simulink model "EPT"  (R2019b)
settings: Solver=FixedStepDiscrete  StartTime=0.0  StopTime=5  FixedStep=0.005  RelTol=1e-3  EnableMultiTasking=on
PreLoadFcn:
  | try, model_open; catch, disp('Error occurred while executing model pre-load callback: model_open.m'); disp('Please assure that the MATLAB working directory is set to the model directory before opening.'); end
InitFcn:
  | try, model_open; catch, end
undefined symbols (not defined in the file or in its folder): Bridge, GCM, H, ln, raptor_get_param_eval, raptor_get_safe_string, raptor_xcp_function
libraries: Raptor_lib x2810, simulink x374, hdlsllib x19
(part 19 of 45)

== system EPT/Foreground_TimeBase_5ms/CAN/CAN3_exec/HyPer9_MCU/TPDO6 ==
  Trigger : TriggerPort  VariantControl=Variant  PortDimensions=1
  Constant : Constant  Value=0.001  OutDataTypeStr=double
  Constant1 : Constant  Value=0.001  OutDataTypeStr=double
  Constant2 : Constant  Value=0.001  OutDataTypeStr=double
  Constant3 : Constant  Value=4  OutDataTypeStr=double
  Constant4 : Constant  Value=4  OutDataTypeStr=double
  Convert_Byte2Data : Subsystem
  Convert_Byte2Data1 : Subsystem
  Convert_Byte2Data2 : Subsystem
  Convert_Byte2Data3 : Subsystem
  Convert_Byte2Data4 : Subsystem
  Demux : Demux  Outputs=8
  raptor_can_rxraw : Raptor_lib/CAN/raptor_can_rxraw  canBus='CAN3'  extendedId=0  showAge=1  id=hex2dec('6A0')  idMask=hex2dec('1FFFFFFF')  mailbox=''  queueSize=1
      settings: SourceProductName=Raptor
  raptor_measurement1 : Raptor_lib/Data Storage/raptor_measurement  paramName='Meas_Motor2_Current'  nameSource=Parameter  calDispType=Number  calEnum={'False', 'True'}  calGain=1.0  calOffset=0.0  calMax=inf  calMin=-inf  calFormat='-1'  calUnit=''  calHelp=''  calAccess=1  calFunction=raptor_xcp_function(gcb)  calVisible=on
      settings: SourceProductName=Raptor
  raptor_measurement2 : Raptor_lib/Data Storage/raptor_measurement  paramName='Meas_Motor1_Current'  nameSource=Parameter  calDispType=Number  calEnum={'False', 'True'}  calGain=1.0  calOffset=0.0  calMax=inf  calMin=-inf  calFormat='-1'  calUnit=''  calHelp=''  calAccess=1  calFunction=raptor_xcp_function(gcb)  calVisible=on
      settings: SourceProductName=Raptor
  raptor_measurement3 : Raptor_lib/Data Storage/raptor_measurement  paramName='Meas_Driver_Output3_Current'  nameSource=Parameter  calDispType=Number  calEnum={'False', 'True'}  calGain=1.0  calOffset=0.0  calMax=inf  calMin=-inf  calFormat='-1'  calUnit=''  calHelp=''  calAccess=1  calFunction=raptor_xcp_function(gcb)  calVisible=on
      settings: SourceProductName=Raptor
  raptor_measurement4 : Raptor_lib/Data Storage/raptor_measurement  paramName='Meas_Driver_Output2_Current'  nameSource=Parameter  calDispType=Number  calEnum={'False', 'True'}  calGain=1.0  calOffset=0.0  calMax=inf  calMin=-inf  calFormat='-1'  calUnit=''  calHelp=''  calAccess=1  calFunction=raptor_xcp_function(gcb)  calVisible=on
      settings: SourceProductName=Raptor
  raptor_measurement5 : Raptor_lib/Data Storage/raptor_measurement  paramName='Meas_Driver_Output1_Current'  nameSource=Parameter  calDispType=Number  calEnum={'False', 'True'}  calGain=1.0  calOffset=0.0  calMax=inf  calMin=-inf  calFormat='-1'  calUnit=''  calHelp=''  calAccess=1  calFunction=raptor_xcp_function(gcb)  calVisible=on
      settings: SourceProductName=Raptor
  wires:
  Constant1/1 -> Convert_Byte2Data1/4(Factor)
  Constant/1 -> Convert_Byte2Data/4(Factor)
  Demux/3 -> Convert_Byte2Data1/1(LowByte)
  Demux/4 -> Convert_Byte2Data1/2(HighByte)
  Convert_Byte2Data1/1(Data) -> raptor_measurement4/1
  Convert_Byte2Data/1(Data) -> raptor_measurement5/1
  Demux/2 -> Convert_Byte2Data/2(HighByte)
  Demux/1 -> Convert_Byte2Data/1(LowByte)
  raptor_can_rxraw/5 -> Demux/1
  Convert_Byte2Data2/1(Data) -> raptor_measurement3/1
  Demux/6 -> Convert_Byte2Data2/2(HighByte)
  Demux/5 -> Convert_Byte2Data2/1(LowByte)
  Constant2/1 -> Convert_Byte2Data2/4(Factor)
  Convert_Byte2Data3/1(Data) -> raptor_measurement2/1
  Convert_Byte2Data4/1(Data) -> raptor_measurement1/1
  Demux/7 -> Convert_Byte2Data3/2(LowByte)
  Demux/8 -> Convert_Byte2Data4/2(LowByte)
  Constant3/1 -> Convert_Byte2Data3/3(Factor)
  Constant4/1 -> Convert_Byte2Data4/3(Factor)

== system EPT/Foreground_TimeBase_5ms/CAN/CAN3_exec/OBC/CountTrigger ==
  Counter : Inport
  Constant1 : Constant  Value=0
  Constant3 : Constant
  CycleTrigger : Subsystem
  Switch : Switch  Threshold=1
  Unit Delay : UnitDelay  SampleTime=-1  HasFrameUpgradeWarning=on
  Tirgger : Outport  VectorParamsAs1DForOutWhenUnconnected=off
  wires:
  Switch/1 -> CycleTrigger/1(In1)
  Constant3/1 -> Switch/3
  Constant1/1 -> Switch/1
  Counter/1 -> CycleTrigger/2(In2)
  CycleTrigger/1(Trigger) -> Tirgger/1, Unit Delay/1
  Unit Delay/1 -> Switch/2

== system EPT/Foreground_TimeBase_5ms/CAN/CAN3_exec/OBC/CountTrigger1 ==
  Counter : Inport
  Constant1 : Constant  Value=0
  Constant3 : Constant
  CycleTrigger : Subsystem
  Switch : Switch  Threshold=1
  Unit Delay : UnitDelay  SampleTime=-1  HasFrameUpgradeWarning=on
  Tirgger : Outport  VectorParamsAs1DForOutWhenUnconnected=off
  wires:
  Switch/1 -> CycleTrigger/1(In1)
  Constant3/1 -> Switch/3
  Constant1/1 -> Switch/1
  Counter/1 -> CycleTrigger/2(In2)
  CycleTrigger/1(Trigger) -> Tirgger/1, Unit Delay/1
  Unit Delay/1 -> Switch/2

== system EPT/Foreground_TimeBase_5ms/CAN/CAN3_exec/OBC/OBC ==
  Rx_Time : Inport
  Tx_Time : Inport  Port=2
  OBC_Rx : Subsystem
  OBC_Tx : Subsystem
  wires:
  Rx_Time/1 -> OBC_Rx/Trigger
  Tx_Time/1 -> OBC_Tx/Trigger

== system EPT/Foreground_TimeBase_5ms/CAN/CAN3_exec/PWCU_GENERATOR/CountTrigger ==
  Counter : Inport
  Constant1 : Constant  Value=0
  Constant3 : Constant
  CycleTrigger : Subsystem
  Switch : Switch  Threshold=1
  Unit Delay : UnitDelay  SampleTime=-1  HasFrameUpgradeWarning=on
  Tirgger : Outport  VectorParamsAs1DForOutWhenUnconnected=off
  wires:
  Unit Delay/1 -> Switch/2
  CycleTrigger/1(Trigger) -> Unit Delay/1, Tirgger/1
  Counter/1 -> CycleTrigger/2(In2)
  Constant1/1 -> Switch/1
  Constant3/1 -> Switch/3
  Switch/1 -> CycleTrigger/1(In1)

== system EPT/Foreground_TimeBase_5ms/CAN/CAN3_exec/PWCU_GENERATOR/CountTrigger1 ==
  Counter : Inport
  Constant1 : Constant  Value=0
  Constant3 : Constant
  CycleTrigger : Subsystem
  Switch : Switch  Threshold=1
  Unit Delay : UnitDelay  SampleTime=-1  HasFrameUpgradeWarning=on
  Tirgger : Outport  VectorParamsAs1DForOutWhenUnconnected=off
  wires:
  Unit Delay/1 -> Switch/2
  CycleTrigger/1(Trigger) -> Unit Delay/1, Tirgger/1
  Counter/1 -> CycleTrigger/2(In2)
  Constant1/1 -> Switch/1
  Constant3/1 -> Switch/3
  Switch/1 -> CycleTrigger/1(In1)

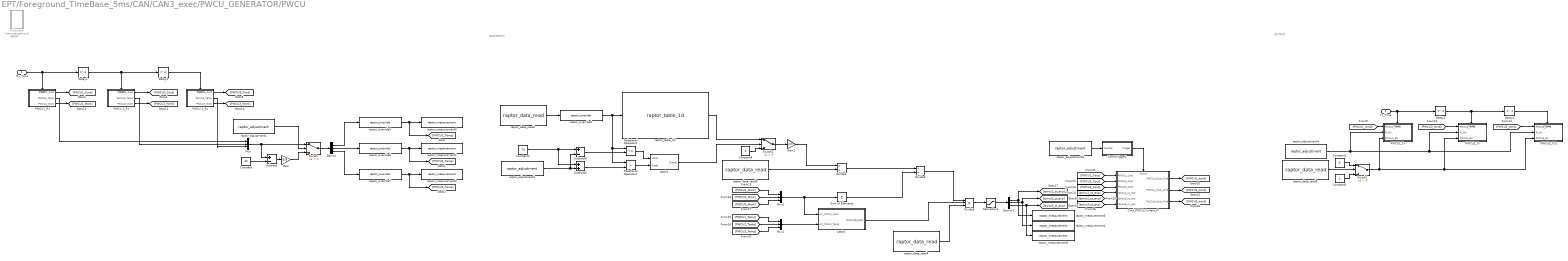
== system EPT/Foreground_TimeBase_5ms/CAN/CAN3_exec/PWCU_GENERATOR/PWCU ==
  note: INPUT
  note: OUTPUT
  note: Applictation
  Rx_Time : Inport
  Tx_Time : Inport  Port=2
  "Cmd_PWCU_Current_PI " : Subsystem
  Constant : Constant  Value=32
  Constant1 : Constant  Value=0
  Constant2 : Constant  Value=70
  Constant3 : Constant
  Constant4 : Constant  Value=0
  CountTrigger1 : Subsystem
  Delay{1..4} (4 alike) : Delay  DelayLength=1
  Demux : Demux  Outputs=3
  Demux1 : Demux  Outputs=3
  Divide3 : Product  Inputs=*/
  Divide4 : Product  Inputs=*/
  Divide5 : Product  Inputs=***
  Gain : Gain  Gain=5/9
  Gain1 : Gain  Gain=1000
  Latch1 : Subsystem
  Latch2 : Subsystem
  Mux : Mux  Inputs=3
  Mux1 : Mux  Inputs=3
  Mux2 : Mux  Inputs=3
  PWCU 2_Rx : Subsystem
  PWCU 3_Rx : Subsystem
  PWCU1_Rx : Subsystem
  PWCU1_Tx : Subsystem
  PWCU2_Tx : Subsystem
  PWCU3_Tx3 : Subsystem
  Relational Operator2 : RelationalOperator  Operator=>  OutDataTypeStr=boolean  RndMeth=Simplest
  Relational Operator4 : RelationalOperator  Operator=<=  OutDataTypeStr=boolean  RndMeth=Simplest
  Saturation1 : Saturate  UpperLimit=20  LowerLimit=0
  Subsystem : Subsystem  Commented=on
  Subtract : Sum  Inputs=+-
  Subtract5 : Sum
  Subtract6 : Sum  Inputs=+-
  Sum of Elements : Sum  Inputs=+
  Switch : Switch  Criteria=u2 > Threshold
  Switch1 : Switch  Criteria=u2 > Threshold
  Switch2 : Switch  Criteria=u2 > Threshold
  raptor_adjustment1 : Raptor_lib/Data Storage/raptor_adjustment  paramName='Cal_Degree_Celsius'  nameSource=Parameter  initValue=0  dataType=boolean  storage=Calibration  calDispType=Number  calEnum={'False', 'True'}  calGain=1.0  calOffset=0.0  calMax=inf  calMin=-inf  calFormat='-1'  calUnit=''  calHelp=''  calAccess=1  calFunction=raptor_xcp_function(gcb)  calDispHeaders=off  calColHeaders={'Col1' 'Col2' 'Col3'}  calRowHeaders={'Row1' 'Row2' 'Row3'}
      settings: SourceProductName=Raptor
  raptor_adjustment16 : Raptor_lib/Data Storage/raptor_adjustment  paramName='PWCU_PI_Time'  nameSource=Parameter  initValue=30  dataType=double  storage=Calibration  calDispType=Number  calEnum={'False', 'True'}  calGain=1.0  calOffset=0.0  calMax=inf  calMin=-inf  calFormat='-1'  calUnit=''  calHelp=''  calAccess=1  calFunction=raptor_xcp_function(gcb)  calDispHeaders=off  calColHeaders={'Col1' 'Col2' 'Col3'}  calRowHeaders={'Row1' 'Row2' 'Row3'}
      settings: SourceProductName=Raptor
  raptor_adjustment2 : Raptor_lib/Data Storage/raptor_adjustment  paramName='Cal_RSOC_GENERATOR_Limit_error'  nameSource=Parameter  initValue=1  dataType=double  storage=Calibration  calDispType=Number  calEnum={'False', 'True'}  calGain=1.0  calOffset=0.0  calMax=inf  calMin=-inf  calFormat='-1'  calUnit=''  calHelp=''  calAccess=1  calFunction=raptor_xcp_function(gcb)  calDispHeaders=off  calColHeaders={'Col1' 'Col2' 'Col3'}  calRowHeaders={'Row1' 'Row2' 'Row3'}
      settings: SourceProductName=Raptor
  raptor_adjustment4 : Raptor_lib/Data Storage/raptor_adjustment  paramName='Cal_SWU_PI_On'  nameSource=Parameter  initValue=1  dataType=boolean  storage=Calibration  calDispType=Number  calEnum={'False', 'True'}  calGain=1.0  calOffset=0.0  calMax=inf  calMin=-inf  calFormat='-1'  calUnit=''  calHelp=''  calAccess=1  calFunction=raptor_xcp_function(gcb)  calDispHeaders=off  calColHeaders={'Col1' 'Col2' 'Col3'}  calRowHeaders={'Row1' 'Row2' 'Row3'}
      settings: SourceProductName=Raptor
  raptor_data_read3 : Raptor_lib/Data Storage/raptor_data_read  dataName='EPT_BPOBU_SOC'  dataShape=Scalar  idxSource=Input  idxRow=1  idxCol=1
      settings: SourceProductName=Raptor
  raptor_data_read4 : Raptor_lib/Data Storage/raptor_data_read  dataName='Ft_CHG_Vcell'  dataShape=Scalar  idxSource=Input  idxRow=1  idxCol=1
      settings: SourceProductName=Raptor
  raptor_data_read5 : Raptor_lib/Data Storage/raptor_data_read  dataName='EPT_HV_BUS_VOLT'  dataShape=Scalar  idxSource=Input  idxRow=1  idxCol=1
      settings: SourceProductName=Raptor
  raptor_data_read8 : Raptor_lib/Data Storage/raptor_data_read  dataName='Relay_BMS_SWU'  dataShape=Scalar  idxSource=Input  idxRow=1  idxCol=1
      settings: SourceProductName=Raptor
  raptor_measurement1 : Raptor_lib/Data Storage/raptor_measurement  paramName='Read_PWCU2_Temp'  nameSource=Parameter  calDispType=Number  calEnum={'False', 'True'}  calGain=1.0  calOffset=0.0  calMax=inf  calMin=-inf  calFormat='-1'  calUnit=''  calHelp=''  calAccess=1  calFunction=raptor_xcp_function(gcb)  calVisible=on
      settings: SourceProductName=Raptor
  raptor_measurement2 : Raptor_lib/Data Storage/raptor_measurement  paramName='Read_PWCU3_Temp'  nameSource=Parameter  calDispType=Number  calEnum={'False', 'True'}  calGain=1.0  calOffset=0.0  calMax=inf  calMin=-inf  calFormat='-1'  calUnit=''  calHelp=''  calAccess=1  calFunction=raptor_xcp_function(gcb)  calVisible=on
      settings: SourceProductName=Raptor
  raptor_measurement3 : Raptor_lib/Data Storage/raptor_measurement  paramName='Ipwcu3_cc_exp'  nameSource=Parameter  calDispType=Number  calEnum={'False', 'True'}  calGain=1.0  calOffset=0.0  calMax=inf  calMin=-inf  calFormat='-1'  calUnit=''  calHelp=''  calAccess=1  calFunction=raptor_xcp_function(gcb)  calVisible=on
      settings: SourceProductName=Raptor
  raptor_measurement4 : Raptor_lib/Data Storage/raptor_measurement  paramName='Ipwcu2_cc_exp'  nameSource=Parameter  calDispType=Number  calEnum={'False', 'True'}  calGain=1.0  calOffset=0.0  calMax=inf  calMin=-inf  calFormat='-1'  calUnit=''  calHelp=''  calAccess=1  calFunction=raptor_xcp_function(gcb)  calVisible=on
      settings: SourceProductName=Raptor
  raptor_measurement5 : Raptor_lib/Data Storage/raptor_measurement  paramName='Ipwcu1_cc_exp'  nameSource=Parameter  calDispType=Number  calEnum={'False', 'True'}  calGain=1.0  calOffset=0.0  calMax=inf  calMin=-inf  calFormat='-1'  calUnit=''  calHelp=''  calAccess=1  calFunction=raptor_xcp_function(gcb)  calVisible=on
      settings: SourceProductName=Raptor
  raptor_measurement6 : Raptor_lib/Data Storage/raptor_measurement  paramName='Read_PWCU1_Temp'  nameSource=Parameter  calDispType=Number  calEnum={'False', 'True'}  calGain=1.0  calOffset=0.0  calMax=inf  calMin=-inf  calFormat='-1'  calUnit=''  calHelp=''  calAccess=1  calFunction=raptor_xcp_function(gcb)  calVisible=on
      settings: SourceProductName=Raptor
  raptor_override4 : Raptor_lib/Data Storage/raptor_override  paramName='Cal_PWCU_EPT_BPOBU_SOC'  nameSource=Parameter  measurement=None  calDispType=Number  calEnum={'False', 'True'}  calGain=1.0  calOffset=0.0  calMax=inf  calMin=-inf  calFormat='-1'  calUnit=''  calHelp=''  calAccess=1  calFunction=[raptor_xcp_function(gcb) '|' raptor_get_param_eval(gcb, 'paramName') '_Override']
      settings: SourceProductName=Raptor
  raptor_override5 : Raptor_lib/Data Storage/raptor_override  paramName='Cal_PWCU1_Temp'  nameSource=Parameter  measurement=None  calDispType=Number  calEnum={'False', 'True'}  calGain=1.0  calOffset=0.0  calMax=inf  calMin=-inf  calFormat='-1'  calUnit=''  calHelp=''  calAccess=1  calFunction=[raptor_xcp_function(gcb) '|' raptor_get_param_eval(gcb, 'paramName') '_Override']
      settings: SourceProductName=Raptor
  raptor_override6 : Raptor_lib/Data Storage/raptor_override  paramName='Cal_PWCU2_Temp'  nameSource=Parameter  measurement=None  calDispType=Number  calEnum={'False', 'True'}  calGain=1.0  calOffset=0.0  calMax=inf  calMin=-inf  calFormat='-1'  calUnit=''  calHelp=''  calAccess=1  calFunction=[raptor_xcp_function(gcb) '|' raptor_get_param_eval(gcb, 'paramName') '_Override']
      settings: SourceProductName=Raptor
  raptor_override7 : Raptor_lib/Data Storage/raptor_override  paramName='Cal_PWCU3_Temp'  nameSource=Parameter  measurement=None  calDispType=Number  calEnum={'False', 'True'}  calGain=1.0  calOffset=0.0  calMax=inf  calMin=-inf  calFormat='-1'  calUnit=''  calHelp=''  calAccess=1  calFunction=[raptor_xcp_function(gcb) '|' raptor_get_param_eval(gcb, 'paramName') '_Override']
      settings: SourceProductName=Raptor
  raptor_table_1d : Raptor_lib/Table Lookup/raptor_table_1d  dataName='OBU_SOC2GENERATOR_PW'  initValue=[6 6 4 4 4 2]  dataType=double  storage=Calibration  initValueX=[0 50 58 60 62 70]  dataTypeXY=double  storageXY=Calibration  calVisible=on  showTable=on  calGain=1.0  calOffset=0.0  calMax=Inf  calMin=-Inf  calFormat='-1'  calUnit=''  calHelp=''  showBreakpoint=on  dataNameX=[]  calGainX=1.0  calOffsetX=0.0  calMaxX=Inf  calMinX=-Inf  calFormatX='-1'  calUnitX=''  calHelpX=''  calAccess=1  calFunction=raptor_xcp_function(gcb)  measureEnable=off  mName=[raptor_get_param_eval(gcb,'dataName'), '_Output']
      settings: SourceProductName=Raptor
  wires:
  raptor_adjustment4/1 -> PWCU3_Tx3/2(PI_On), PWCU2_Tx/2(PI_On), PWCU1_Tx/2(PI_On)
  Tx_Time/1 -> Delay2/1, PWCU1_Tx/Trigger
  Delay2/1 -> Delay4/1, PWCU2_Tx/Trigger
  Rx_Time/1 -> Delay1/1, PWCU1_Rx/Trigger
  Delay1/1 -> Delay3/1, PWCU 2_Rx/Trigger
  Delay3/1 -> PWCU 3_Rx/Trigger
  PWCU1_Rx/2("PWCU1_Temp ") -> Mux/1
  PWCU 2_Rx/2("PWCU2_Temp ") -> Mux/2
  PWCU1_Rx/1("PWCU1_Cout ") -> [PWCU1_Cout]
  PWCU 2_Rx/1("PWCU2_Cout ") -> [PWCU2_Cout]
  PWCU 3_Rx/1("PWCU3_Cout ") -> [PWCU3_Cout]
  Delay4/1 -> PWCU3_Tx3/Trigger
  [PWCU1_Icmd] -> PWCU1_Tx/1(PWCU1_Icmd)
  [PWCU2_Icmd] -> PWCU2_Tx/1(PWCU2_Icmd)
  [PWCU3_Icmd] -> PWCU3_Tx3/1(PWCU3_Icmd)
  PWCU 2_Rx/3(PWCU2_Work) -> [PWCU2_Work]
  PWCU1_Rx/3(PWCU1_Work) -> [PWCU1_Work]
  PWCU 3_Rx/3(PWCU3_Work) -> [PWCU3_Work]
  raptor_data_read8/1 -> Switch1/2
  Constant1/1 -> Switch1/1
  Switch1/1 -> PWCU1_Tx/3(PWCU1_EN), PWCU3_Tx3/3(PWCU3_EN), PWCU2_Tx/3(PWCU2_EN)
  Constant3/1 -> Switch1/3
  [PWCU3_Temp] -> Mux1/3
  [PWCU2_Temp] -> Mux1/2
  [PWCU1_Temp] -> Mux1/1
  raptor_data_read4/1 -> Divide5/3
  Demux1/2 -> [Ipwcu2_cc_exp], raptor_measurement4/1
  Demux1/3 -> [Ipwcu3_cc_exp], raptor_measurement3/1
  Demux1/1 -> raptor_measurement5/1, [Ipwcu1_cc_exp]
  Saturation1/1 -> Demux1/1
  [PWCU1_Work] -> Mux2/1
  "Cmd_PWCU_Current_PI "/3(PWCU3_Cout_Cmd) -> [PWCU3_Icmd]
  "Cmd_PWCU_Current_PI "/2(PWCU2_Cout_Cmd) -> [PWCU2_Icmd]
  "Cmd_PWCU_Current_PI "/1(PWCU1_Cout_Cmd) -> [PWCU1_Icmd]
  Divide5/1 -> Saturation1/1
  [Ipwcu3_cc_exp] -> "Cmd_PWCU_Current_PI "/6(Ipwcu3_cc_exp)
  [Ipwcu2_cc_exp] -> "Cmd_PWCU_Current_PI "/5(Ipwcu2_cc_exp)
  [PWCU3_Cout] -> "Cmd_PWCU_Current_PI "/3(PWCU3_Cout)
  [Ipwcu1_cc_exp] -> "Cmd_PWCU_Current_PI "/4(Ipwcu1_cc_exp)
  [PWCU2_Cout] -> "Cmd_PWCU_Current_PI "/2(PWCU2_Cout)
  [PWCU1_Cout] -> "Cmd_PWCU_Current_PI "/1(PWCU1_Cout)
  Divide4/1 -> Divide5/1
  Divide3/1 -> Divide4/1
  Gain1/1 -> Divide3/1
  Mux1/1 -> Latch1/2(Arr_PWCU_Temp)
  raptor_data_read3/1 -> raptor_override4/1
  raptor_adjustment16/1 -> CountTrigger1/1(Counter)
  CountTrigger1/1(Tirgger) -> "Cmd_PWCU_Current_PI "/Enable
  PWCU 3_Rx/2("PWCU3_Temp ") -> Mux/3
  raptor_adjustment1/1 -> Switch/2
  raptor_override7/1 -> [PWCU3_Temp], raptor_measurement2/1
  Subtract/1 -> Gain/1
  Mux/1 -> Subtract/1, Switch/1
  Constant/1 -> Subtract/2
  Gain/1 -> Switch/3
  Switch/1 -> Demux/1
  Demux/1 -> raptor_override5/1
  Demux/2 -> raptor_override6/1
  Demux/3 -> raptor_override7/1
  raptor_override6/1 -> [PWCU2_Temp], raptor_measurement1/1
  raptor_override5/1 -> [PWCU1_Temp], raptor_measurement6/1
  Subtract5/1 -> Relational Operator2/2
  Relational Operator4/1 -> Latch2/1(Latch)
  Constant2/1 -> Subtract6/1, Subtract5/1
  Relational Operator2/1 -> Latch2/2(Reset)
  raptor_override4/1 -> Relational Operator4/1, Relational Operator2/1, raptor_table_1d/1
  raptor_adjustment2/1 -> Subtract5/2, Subtract6/2
  Subtract6/1 -> Relational Operator4/2
  Latch2/1(Output) -> Switch2/2
  raptor_table_1d/1 -> Switch2/1
  Switch2/1 -> Gain1/1
  Constant4/1 -> Switch2/3
  raptor_data_read5/1 -> Divide3/2
  [PWCU2_Work] -> Mux2/2
  [PWCU3_Work] -> Mux2/3
  Mux2/1 -> Sum of Elements/1, Latch1/1(Arr_PWCU_Work)
  Sum of Elements/1 -> Divide4/2
  Latch1/1(PWCUTemp2Ft) -> Divide5/2

== system EPT/Foreground_TimeBase_5ms/CAN/CAN3_exec/SEVCON_MCU /CountTrigger1 ==
  Counter : Inport
  Constant1 : Constant  Value=0
  Constant3 : Constant
  CycleTrigger : Subsystem
  Switch : Switch  Threshold=1
  Unit Delay1 : UnitDelay  SampleTime=-1  HasFrameUpgradeWarning=on
  Unit Delay2 : UnitDelay  SampleTime=-1  HasFrameUpgradeWarning=on
  Tirgger : Outport  VectorParamsAs1DForOutWhenUnconnected=off
  wires:
  Unit Delay2/1 -> Tirgger/1
  Unit Delay1/1 -> CycleTrigger/1(In1)
  CycleTrigger/1(Trigger) -> Unit Delay2/1, Switch/2
  Counter/1 -> CycleTrigger/2(In2)
  Constant1/1 -> Switch/1
  Constant3/1 -> Switch/3
  Switch/1 -> Unit Delay1/1

== system EPT/Foreground_TimeBase_5ms/CAN/CAN3_exec/SEVCON_MCU /CountTrigger2 ==
  Counter : Inport
  Constant1 : Constant  Value=0
  Constant3 : Constant
  CycleTrigger : Subsystem
  Switch : Switch  Threshold=1
  Unit Delay1 : UnitDelay  SampleTime=-1  HasFrameUpgradeWarning=on
  Unit Delay2 : UnitDelay  SampleTime=-1  HasFrameUpgradeWarning=on
  Tirgger : Outport  VectorParamsAs1DForOutWhenUnconnected=off
  wires:
  Unit Delay2/1 -> Tirgger/1
  Unit Delay1/1 -> CycleTrigger/1(In1)
  CycleTrigger/1(Trigger) -> Unit Delay2/1, Switch/2
  Counter/1 -> CycleTrigger/2(In2)
  Constant1/1 -> Switch/1
  Constant3/1 -> Switch/3
  Switch/1 -> Unit Delay1/1

== system EPT/Foreground_TimeBase_5ms/CAN/CAN3_exec/SEVCON_MCU /SEVCON_Error_Code ==
  note: If any of bytes b5-b7 are not 0x00 means error is set.
      | If bytes b5-b7 are all 00 it means the error is reset.
  Compare To Constant : simulink/Logic and Bit Operations/Compare To Constant  relop=>  const=3.0  OutDataTypeStr=boolean
  Constant : Constant
  Constant1 : Constant  Value=0
  Convert_Byte2Data1 : Subsystem
  Convert_Byte2Data2 : Subsystem
  Data Type Conversion : DataTypeConversion  OutDataTypeStr=double
  Data Type Conversion1 : DataTypeConversion  OutDataTypeStr=uint8
  Data Type Conversion2 : DataTypeConversion  OutDataTypeStr=uint16
  Data Type Conversion3 : DataTypeConversion  OutDataTypeStr=int16
  Demux : Demux  Outputs=8
  Demux1 : Demux  Outputs=2
  EPT_MCU_FAULT_LEVEL : Subsystem
  "Error_Cause " : Subsystem
  IsNonZero : simulink/Logic and Bit Operations/Compare To Zero  relop=~=  OutDataTypeStr=boolean
  IsNonZero1 : simulink/Logic and Bit Operations/Compare To Zero  relop=~=  OutDataTypeStr=boolean
  IsNonZero2 : simulink/Logic and Bit Operations/Compare To Zero  relop=~=  OutDataTypeStr=boolean
  Logical Operator : Logic  Operator=OR  Inputs=3  AllPortsSameDT=off  OutDataTypeStr=boolean
  Logical Operator1 : Logic  Operator=OR  AllPortsSameDT=off  OutDataTypeStr=boolean
  Logical Operator2 : Logic  Inputs=3  AllPortsSameDT=off  OutDataTypeStr=boolean
  Logical Operator4 : Logic  AllPortsSameDT=off  OutDataTypeStr=boolean
  Mux : Mux  Inputs=2
  NOT : Logic  Operator=NOT  IconShape=distinctive  AllPortsSameDT=off  OutDataTypeStr=boolean
  Switch : Switch  Criteria=u2 > Threshold
  raptor_can_rxraw1 : Raptor_lib/CAN/raptor_can_rxraw  canBus='CAN3'  extendedId=0  showAge=1  id=hex2dec('081')  idMask=hex2dec('1FFFFFFF')  mailbox=''  queueSize=1
      settings: SourceProductName=Raptor
  raptor_data_def : Raptor_lib/Data Storage/raptor_data_def  dataName='MCU_CANopen_Error_Code'  initValue=0  dataType=double  storage=Volatile (RAM)  calVisible=on  calType=Adjustment  calDispType=Number  calEnum={'False', 'True'}  calGain=1.0  calOffset=0  calMin=-inf  calMax=inf  calFormat='-1'  calUnit=''  calHelp=''  calAccess=1  calFunction=raptor_xcp_function(gcb)  calDispHeaders=off  calColHeaders={'Col1' 'Col2' 'Col3'}  calRowHeaders={'Row1' 'Row2' 'Row3'}
      settings: SourceProductName=Raptor
  raptor_data_def1 : Raptor_lib/Data Storage/raptor_data_def  dataName='EPT_MCU_FAULT_CAUSE'  initValue=0  dataType=uint8  storage=Volatile (RAM)  calVisible=on  calType=Measurement  calDispType=Number  calEnum={'False', 'True'}  calGain=1.0  calOffset=0  calMin=-inf  calMax=inf  calFormat='-1'  calUnit=''  calHelp=''  calAccess=1  calFunction=raptor_xcp_function(gcb)  calDispHeaders=off  calColHeaders={'Col1' 'Col2' 'Col3'}  calRowHeaders={'Row1' 'Row2' 'Row3'}
      settings: SourceProductName=Raptor
  raptor_data_def2 : Raptor_lib/Data Storage/raptor_data_def  dataName='EPT_MCU_FAULT_ID'  initValue=0  dataType=uint16  storage=Volatile (RAM)  calVisible=on  calType=Measurement  calDispType=Number  calEnum={'False', 'True'}  calGain=1.0  calOffset=0  calMin=-inf  calMax=inf  calFormat='-1'  calUnit=''  calHelp=''  calAccess=1  calFunction=raptor_xcp_function(gcb)  calDispHeaders=off  calColHeaders={'Col1' 'Col2' 'Col3'}  calRowHeaders={'Row1' 'Row2' 'Row3'}
      settings: SourceProductName=Raptor
  raptor_data_read : Raptor_lib/Data Storage/raptor_data_read  dataName='EPT_MCU_FAULT_LEVEL'  dataShape=Scalar  idxSource=Input  idxRow=1  idxCol=1
      settings: SourceProductName=Raptor
  raptor_data_read1 : Raptor_lib/Data Storage/raptor_data_read  dataName='CAN_Fault_MCU'  dataShape=Scalar  idxSource=Input  idxRow=1  idxCol=1
      settings: SourceProductName=Raptor
  raptor_data_read2 : Raptor_lib/Data Storage/raptor_data_read  dataName='Relay_MCU'  dataShape=Scalar  idxSource=Input  idxRow=1  idxCol=1
      settings: SourceProductName=Raptor
  raptor_data_write : Raptor_lib/Data Storage/raptor_data_write  dataName='MCU_CANopen_Error_Code'  dataShape=Scalar  idxSource=Input Port  idxRow=1  idxCol=1
      settings: SourceProductName=Raptor
  raptor_data_write1 : Raptor_lib/Data Storage/raptor_data_write  dataName='EPT_MCU_FAULT_CAUSE'  dataShape=Scalar  idxSource=Input Port  idxRow=1  idxCol=1
      settings: SourceProductName=Raptor
  raptor_data_write2 : Raptor_lib/Data Storage/raptor_data_write  dataName='EPT_MCU_FAULT_ID'  dataShape=Scalar  idxSource=Input Port  idxRow=1  idxCol=1
      settings: SourceProductName=Raptor
  raptor_data_write3 : Raptor_lib/Data Storage/raptor_data_write  dataName='EPT_MOTOR_FAULT'  dataShape=Scalar  idxSource=Input Port  idxRow=1  idxCol=1
      settings: SourceProductName=Raptor
  wires:
  Demux/1 -> Convert_Byte2Data1/1(LowByte)
  Constant/1 -> Convert_Byte2Data2/3(Factor), Convert_Byte2Data1/3(Factor)
  raptor_can_rxraw1/5 -> Demux/1
  Demux/2 -> Convert_Byte2Data1/2(HighByte)
  Constant1/1 -> Convert_Byte2Data2/4(Offset), Convert_Byte2Data1/4(Offset)
  Demux/4 -> Convert_Byte2Data2/1(LowByte)
  Demux/5 -> Convert_Byte2Data2/2(HighByte)
  Data Type Conversion/1 -> raptor_data_write/1
  Data Type Conversion1/1 -> raptor_data_write1/1
  Data Type Conversion2/1 -> raptor_data_write2/1
  Demux/7 -> IsNonZero1/1
  Demux/8 -> IsNonZero2/1
  Demux/6 -> IsNonZero/1
  IsNonZero1/1 -> Logical Operator/2
  IsNonZero/1 -> Logical Operator/1
  IsNonZero2/1 -> Logical Operator/3
  raptor_data_read1/1 -> Logical Operator1/2, NOT/1
  Logical Operator/1 -> Logical Operator2/1
  Logical Operator4/1 -> Logical Operator2/2
  Demux/3 -> Data Type Conversion3/1
  Convert_Byte2Data1/1(Data(int16)) -> Mux/1
  Mux/1 -> Switch/1
  Switch/1 -> Demux1/1
  Demux1/2 -> Data Type Conversion1/1
  Demux1/1 -> Data Type Conversion/1
  raptor_data_read/1 -> Compare To Constant/1
  Compare To Constant/1 -> Logical Operator2/3
  Data Type Conversion3/1 -> Mux/2
  raptor_data_read2/1 -> Logical Operator4/1
  NOT/1 -> Logical Operator4/2
  Convert_Byte2Data2/1(Data(int16)) -> Data Type Conversion2/1
  Logical Operator1/1 -> raptor_data_write3/1
  Logical Operator2/1 -> Switch/2, Logical Operator1/1

== system EPT/Foreground_TimeBase_5ms/CAN/CAN3_exec/SEVCON_MCU /SEVCON_RX_0X220_20ms ==
  Trigger : TriggerPort  VariantControl=Variant  PortDimensions=1
  Add : Sum
  Data Type Conversion : DataTypeConversion
  Data Type Conversion1 : DataTypeConversion  OutDataTypeStr=uint8
  Data Type Conversion2 : DataTypeConversion  OutDataTypeStr=uint8
  Shift Arithmetic : ArithShift  BitShiftNumber=1  BitShiftDirection=Left
  raptor_can_rxmsg : Raptor_lib/CAN/raptor_can_rxmsg  canDefinition=struct('dbcFile', 'SEVCON_Controller_CANopen.dbc','message', 'Read2','comment', '','signals', {{'Read_Handbrake_Switch','Read_Seat_Switch','Read_Reverse_Switch','Read_Forward_Switch','Read_Actual_Torque','Read_Controller_Cap_Voltage','Read_Motor_Temp','Read_Controller_Temp'}},'enabled', [ 1 1 1 1 1 1 1 1;],'canBus', '''CAN3''','messageID', [ 544;],'idMask', [ 536870911;],'payloadMask', [],'payloadValue', [],'period', [ 0;],'mailbox', '''''','queueSize', [ 1;],'label', [ 0;],'ver', [ 2;],'showID', [ 0;],'showRaw', [ 0;],'fill', [ 0;],'editID', [ 0;],'signalOrder', [ 2;])  canBus='CAN3'  mailbox=''  payloadMask=[]  payloadValue=[]  idMask=hex2dec('1FFFFFFF')  queueSize=1  showID=0  label=0  fill=0  id=544  showRaw=0  showAge=1  signalOrder=2  signalInfo={{struct('Name', 'Read_Actual_Torque','Startbit', [ 0;],'SignalSize', [ 16;],'ByteOrder', 'LittleEndian','ValueType', 'SIGNED','Class', 'int16','Signed', [ 1;],'Factor', [ 0.1;],'Offset', [ 0;],'Min', [ 0;],'Max', [ 0;],'Units', '','Comment', '','StartBit', [ 40;]),struct('Name', 'Read_Seat_Switch','Startbit', [ 0;],'SignalSize', [ 1;],'ByteOrder', 'LittleEndian','ValueType', 'UNSIGNED','Class', 'uint8','Signed', [ 0;],'Factor', [ 1;],'Offset', [ 0;],'Min', [ 0;],'Max', [ 0;],'Units', '','Comment', '','StartBit', [ 58;]),struct('Name', 'Read_Reverse_Switch','Startbit', [ 0;],'SignalSize', [ 1;],'ByteOrder', 'LittleEndian','ValueType', 'UNSIGNED','Class', 'uint8','Signed', [ 0;],'Factor', [ 1;],'Offset', [ 0;],'Min', [ 0;],'Max', [ 0;],'Units', '','Comment', '','StartBit', [ 57;]),struct('Name', 'Read_Handbrake_Switch','Startbit', [ 0;],'SignalSize', [ 1;],'ByteOrder', 'LittleEndian','ValueType', 'UNSIGNED','Class', 'uint8','Signed', [ 0;],'Factor', [ 1;],'Offset', [ 0;],'Min', [ 0;],'Max', [ 0;],'Units', '','Comment', '','StartBit', [ 59;]),struct('Name', 'Read_Forward_Switch','Startbit', [ 0;],'SignalSize', [ 1;],'ByteOrder', 'LittleEndian','ValueType', 'UNSIGNED','Class', 'uint8','Signed', [ 0;],'Factor', [ 1;],'Offset', [ 0;],'Min', [ 0;],'Max', [ 0;],'Units', '','Comment', '','StartBit', [ 56;]),struct('Name', 'Read_Motor_Temp','Startbit', [ 0;],'SignalSize', [ 16;],'ByteOrder', 'LittleEndian','ValueType', 'SIGNED','Class', 'int16','Signed', [ 1;],'Factor', [ 1;],'Offset', [ 0;],'Min', [ 0;],'Max', [ 0;],'Units', '','Comment', '','StartBit', [ 8;]),struct('Name', 'Read_Controller_Temp','Startbit', [ 0;],'SignalSize', [ 8;],'ByteOrder', 'LittleEndian','ValueType', 'SIGNED','Class', 'int8','Signed', [ 1;],'Factor', [ 1;],'Offset', [ 0;],'Min', [ 0;],'Max', [ 0;],'Units', '','Comment', '','StartBit', [ 0;]),struct('Name', 'Read_Controller_Cap_Voltage','Startbit', [ 0;],'SignalSize', [ 16;],'ByteOrder', 'LittleEndian','ValueType', 'SIGNED','Class', 'int16','Signed', [ 1;],'Factor', [ 0.0625;],'Offset', [ 0;],'Min', [ 0;],'Max', [ 0;],'Units', '','Comment', '','StartBit', [ 24;])}}
      settings: SourceProductName=Raptor
  raptor_data_def1 : Raptor_lib/Data Storage/raptor_data_def  dataName='Read_Motor_Temp'  initValue=0  dataType=double  storage=Volatile (RAM)  calVisible=on  calType=Adjustment  calDispType=Number  calEnum={'False', 'True'}  calGain=1.0  calOffset=0  calMin=-inf  calMax=inf  calFormat='-1'  calUnit=''  calHelp=''  calAccess=1  calFunction=raptor_xcp_function(gcb)  calDispHeaders=off  calColHeaders={'Col1' 'Col2' 'Col3'}  calRowHeaders={'Row1' 'Row2' 'Row3'}
      settings: SourceProductName=Raptor
  raptor_data_def2 : Raptor_lib/Data Storage/raptor_data_def  dataName='Rx0x220_Age'  initValue=0  dataType=uint16  storage=Volatile (RAM)  calVisible=on  calType=Adjustment  calDispType=Number  calEnum={'False', 'True'}  calGain=1.0  calOffset=0  calMin=-inf  calMax=inf  calFormat='-1'  calUnit=''  calHelp=''  calAccess=1  calFunction=raptor_xcp_function(gcb)  calDispHeaders=off  calColHeaders={'Col1' 'Col2' 'Col3'}  calRowHeaders={'Row1' 'Row2' 'Row3'}
      settings: SourceProductName=Raptor
  raptor_data_def21 : Raptor_lib/Data Storage/raptor_data_def  dataName='Read_Controller_Cap_Voltage'  initValue=0  dataType=double  storage=Volatile (RAM)  calVisible=on  calType=Adjustment  calDispType=Number  calEnum={'False', 'True'}  calGain=1.0  calOffset=0  calMin=-inf  calMax=inf  calFormat='-1'  calUnit=''  calHelp=''  calAccess=1  calFunction=raptor_xcp_function(gcb)  calDispHeaders=off  calColHeaders={'Col1' 'Col2' 'Col3'}  calRowHeaders={'Row1' 'Row2' 'Row3'}
      settings: SourceProductName=Raptor
  raptor_data_def23 : Raptor_lib/Data Storage/raptor_data_def  dataName='Read_Controller_Temp'  initValue=0  dataType=int8  storage=Volatile (RAM)  calVisible=on  calType=Adjustment  calDispType=Number  calEnum={'False', 'True'}  calGain=1.0  calOffset=0  calMin=-inf  calMax=inf  calFormat='-1'  calUnit=''  calHelp=''  calAccess=1  calFunction=raptor_xcp_function(gcb)  calDispHeaders=off  calColHeaders={'Col1' 'Col2' 'Col3'}  calRowHeaders={'Row1' 'Row2' 'Row3'}
      settings: SourceProductName=Raptor
  raptor_data_write : Raptor_lib/Data Storage/raptor_data_write  dataName='EPT_MOTOR_TRQ'  dataShape=Scalar  idxSource=Input Port  idxRow=1  idxCol=1
      settings: SourceProductName=Raptor
  raptor_data_write1 : Raptor_lib/Data Storage/raptor_data_write  dataName='Rx0x220_Age'  dataShape=Scalar  idxSource=Input Port  idxRow=1  idxCol=1
      settings: SourceProductName=Raptor
  raptor_data_write2 : Raptor_lib/Data Storage/raptor_data_write  dataName='Read_Controller_Cap_Voltage'  dataShape=Scalar  idxSource=Input Port  idxRow=1  idxCol=1
      settings: SourceProductName=Raptor
  raptor_data_write3 : Raptor_lib/Data Storage/raptor_data_write  dataName='Read_Motor_Temp'  dataShape=Scalar  idxSource=Input Port  idxRow=1  idxCol=1
      settings: SourceProductName=Raptor
  raptor_data_write4 : Raptor_lib/Data Storage/raptor_data_write  dataName='Read_Controller_Temp'  dataShape=Scalar  idxSource=Input Port  idxRow=1  idxCol=1
      settings: SourceProductName=Raptor
  raptor_data_write5 : Raptor_lib/Data Storage/raptor_data_write  dataName='EPT_GEAR_STA'  dataShape=Scalar  idxSource=Input Port  idxRow=1  idxCol=1
      settings: SourceProductName=Raptor
  raptor_measurement14 : Raptor_lib/Data Storage/raptor_measurement  paramName='Read_Seat_Switch'  nameSource=Parameter  calDispType=Number  calEnum={'False', 'True'}  calGain=1.0  calOffset=0.0  calMax=inf  calMin=-inf  calFormat='-1'  calUnit=''  calHelp=''  calAccess=1  calFunction=raptor_xcp_function(gcb)  calVisible=on
      settings: SourceProductName=Raptor
  raptor_measurement16 : Raptor_lib/Data Storage/raptor_measurement  paramName='Read_Handbrake_Switch'  nameSource=Parameter  calDispType=Number  calEnum={'False', 'True'}  calGain=1.0  calOffset=0.0  calMax=inf  calMin=-inf  calFormat='-1'  calUnit=''  calHelp=''  calAccess=1  calFunction=raptor_xcp_function(gcb)  calVisible=on
      settings: SourceProductName=Raptor
  wires:
  raptor_can_rxmsg/4 -> Data Type Conversion1/1
  raptor_can_rxmsg/2 -> raptor_measurement16/1
  raptor_can_rxmsg/6 -> raptor_data_write/1
  raptor_can_rxmsg/3 -> raptor_measurement14/1
  raptor_can_rxmsg/1 -> raptor_data_write1/1
  raptor_can_rxmsg/9 -> raptor_data_write4/1
  raptor_can_rxmsg/5 -> Data Type Conversion2/1
  raptor_can_rxmsg/7 -> raptor_data_write2/1
  raptor_can_rxmsg/8 -> raptor_data_write3/1
  Shift Arithmetic/1 -> Add/2
  Add/1 -> Data Type Conversion/1
  Data Type Conversion/1 -> raptor_data_write5/1
  Data Type Conversion1/1 -> Add/1
  Data Type Conversion2/1 -> Shift Arithmetic/1

== system EPT/Foreground_TimeBase_5ms/CAN/CAN3_exec/SEVCON_MCU /SEVCON_RX_0X221_20ms ==
  Trigger : TriggerPort  VariantControl=Variant  PortDimensions=1
  raptor_can_rxmsg1 : Raptor_lib/CAN/raptor_can_rxmsg  canDefinition=struct('dbcFile', 'SEVCON_Controller_CANopen.dbc','message', 'Read1','comment', '','signals', {{'Read_Motor_Speed','Read_AC_Motor_Current','Read_AC_Motor_Voltage'}},'enabled', [ 1 1 1;],'canBus', '''CAN3''','messageID', [ 545;],'idMask', [ 536870911;],'payloadMask', [],'payloadValue', [],'period', [ 0;],'mailbox', '''''','queueSize', [ 1;],'label', [ 0;],'ver', [ 2;],'showID', [ 0;],'showRaw', [ 0;],'fill', [ 0;],'editID', [ 0;],'signalOrder', [ 2;])  canBus='CAN3'  mailbox=''  payloadMask=[]  payloadValue=[]  idMask=hex2dec('1FFFFFFF')  queueSize=1  showID=0  label=0  fill=0  id=545  showRaw=0  showAge=1  signalOrder=2  signalInfo={{struct('Name', 'Read_Motor_Speed','Startbit', [ 0;],'SignalSize', [ 32;],'ByteOrder', 'LittleEndian','ValueType', 'SIGNED','Class', 'int32','Signed', [ 1;],'Factor', [ 1;],'Offset', [ 0;],'Min', [ 0;],'Max', [ 0;],'Units', '','Comment', '','StartBit', [ 32;]),struct('Name', 'Read_AC_Motor_Voltage','Startbit', [ 0;],'SignalSize', [ 16;],'ByteOrder', 'LittleEndian','ValueType', 'SIGNED','Class', 'int16','Signed', [ 1;],'Factor', [ 0.0625;],'Offset', [ 0;],'Min', [ 0;],'Max', [ 0;],'Units', '','Comment', '','StartBit', [ 0;]),struct('Name', 'Read_AC_Motor_Current','Startbit', [ 0;],'SignalSize', [ 16;],'ByteOrder', 'LittleEndian','ValueType', 'SIGNED','Class', 'int16','Signed', [ 1;],'Factor', [ 0.0625;],'Offset', [ 0;],'Min', [ 0;],'Max', [ 0;],'Units', '','Comment', '','StartBit', [ 16;])}}
      settings: SourceProductName=Raptor
  raptor_data_def1 : Raptor_lib/Data Storage/raptor_data_def  dataName='Rx0x221_Age'  initValue=0  dataType=uint16  storage=Volatile (RAM)  calVisible=on  calType=Adjustment  calDispType=Number  calEnum={'False', 'True'}  calGain=1.0  calOffset=0  calMin=-inf  calMax=inf  calFormat='-1'  calUnit=''  calHelp=''  calAccess=1  calFunction=raptor_xcp_function(gcb)  calDispHeaders=off  calColHeaders={'Col1' 'Col2' 'Col3'}  calRowHeaders={'Row1' 'Row2' 'Row3'}
      settings: SourceProductName=Raptor
  raptor_data_def2 : Raptor_lib/Data Storage/raptor_data_def  dataName='Read_AC_Motor_Current'  initValue=0  dataType=double  storage=Volatile (RAM)  calVisible=on  calType=Adjustment  calDispType=Number  calEnum={'False', 'True'}  calGain=1.0  calOffset=0  calMin=-inf  calMax=inf  calFormat='-1'  calUnit=''  calHelp=''  calAccess=1  calFunction=raptor_xcp_function(gcb)  calDispHeaders=off  calColHeaders={'Col1' 'Col2' 'Col3'}  calRowHeaders={'Row1' 'Row2' 'Row3'}
      settings: SourceProductName=Raptor
  raptor_data_def21 : Raptor_lib/Data Storage/raptor_data_def  dataName='Read_Motor_Speed'  initValue=0  dataType=double  storage=Volatile (RAM)  calVisible=on  calType=Adjustment  calDispType=Number  calEnum={'False', 'True'}  calGain=1.0  calOffset=0  calMin=-inf  calMax=inf  calFormat='-1'  calUnit=''  calHelp=''  calAccess=1  calFunction=raptor_xcp_function(gcb)  calDispHeaders=off  calColHeaders={'Col1' 'Col2' 'Col3'}  calRowHeaders={'Row1' 'Row2' 'Row3'}
      settings: SourceProductName=Raptor
  raptor_data_write : Raptor_lib/Data Storage/raptor_data_write  dataName='Read_Motor_Speed'  dataShape=Scalar  idxSource=Input Port  idxRow=1  idxCol=1
      settings: SourceProductName=Raptor
  raptor_data_write1 : Raptor_lib/Data Storage/raptor_data_write  dataName='Rx0x221_Age'  dataShape=Scalar  idxSource=Input Port  idxRow=1  idxCol=1
      settings: SourceProductName=Raptor
  raptor_data_write2 : Raptor_lib/Data Storage/raptor_data_write  dataName='Read_AC_Motor_Current'  dataShape=Scalar  idxSource=Input Port  idxRow=1  idxCol=1
      settings: SourceProductName=Raptor
  raptor_measurement3 : Raptor_lib/Data Storage/raptor_measurement  paramName='Read_AC_Motor_Voltage'  nameSource=Parameter  calDispType=Number  calEnum={'False', 'True'}  calGain=1.0  calOffset=0.0  calMax=inf  calMin=-inf  calFormat='-1'  calUnit=''  calHelp=''  calAccess=1  calFunction=raptor_xcp_function(gcb)  calVisible=on
      settings: SourceProductName=Raptor
  wires:
  raptor_can_rxmsg1/4 -> raptor_measurement3/1
  raptor_can_rxmsg1/2 -> raptor_data_write/1
  raptor_can_rxmsg1/3 -> raptor_data_write2/1
  raptor_can_rxmsg1/1 -> raptor_data_write1/1

== system EPT/Foreground_TimeBase_5ms/CAN/CAN3_exec/SEVCON_MCU /SEVCON_RX_0x701_500ms ==
  Trigger : TriggerPort  VariantControl=Variant  PortDimensions=1
  Compare To Constant : simulink/Logic and Bit Operations/Compare To Constant  relop===  const=5  OutDataTypeStr=boolean
  raptor_can_rxmsg1 : Raptor_lib/CAN/raptor_can_rxmsg  canDefinition=struct('dbcFile', 'SEVCON_Controller_CANopen.dbc','message', 'Status','comment', '','signals', {{'Read_MCU_Status'}},'enabled', [ 1;],'canBus', '''CAN3''','messageID', [ 1793;],'idMask', [ 536870911;],'payloadMask', [],'payloadValue', [],'period', [ 0;],'mailbox', '''''','queueSize', [ 1;],'label', [ 0;],'ver', [ 2;],'showID', [ 0;],'showRaw', [ 0;],'fill', [ 0;],'editID', [ 0;],'signalOrder', [ 2;])  canBus='CAN3'  mailbox=''  payloadMask=[]  payloadValue=[]  idMask=hex2dec('1FFFFFFF')  queueSize=1  showID=0  label=0  fill=0  id=1793  showRaw=0  showAge=1  signalOrder=2  signalInfo={{struct('Name', 'Read_MCU_Status','Startbit', [ 0;],'SignalSize', [ 8;],'ByteOrder', 'LittleEndian','ValueType', 'SIGNED','Class', 'int8','Signed', [ 1;],'Factor', [ 1;],'Offset', [ 0;],'Min', [ 0;],'Max', [ 0;],'Units', '','Comment', '','StartBit', [ 0;])}}
      settings: SourceProductName=Raptor
  raptor_data_def1 : Raptor_lib/Data Storage/raptor_data_def  dataName='Rx0x701_Age'  initValue=0  dataType=uint16  storage=Volatile (RAM)  calVisible=on  calType=Adjustment  calDispType=Number  calEnum={'False', 'True'}  calGain=1.0  calOffset=0  calMin=-inf  calMax=inf  calFormat='-1'  calUnit=''  calHelp=''  calAccess=1  calFunction=raptor_xcp_function(gcb)  calDispHeaders=off  calColHeaders={'Col1' 'Col2' 'Col3'}  calRowHeaders={'Row1' 'Row2' 'Row3'}
      settings: SourceProductName=Raptor
  raptor_data_def2 : Raptor_lib/Data Storage/raptor_data_def  dataName='MCU_InitFinishFlag'  initValue=0  dataType=boolean  storage=Volatile (RAM)  calVisible=on  calType=Adjustment  calDispType=Number  calEnum={'False', 'True'}  calGain=1.0  calOffset=0  calMin=-inf  calMax=inf  calFormat='-1'  calUnit=''  calHelp=''  calAccess=1  calFunction=raptor_xcp_function(gcb)  calDispHeaders=off  calColHeaders={'Col1' 'Col2' 'Col3'}  calRowHeaders={'Row1' 'Row2' 'Row3'}
      settings: SourceProductName=Raptor
  raptor_data_def21 : Raptor_lib/Data Storage/raptor_data_def  dataName='Read_MCU_Status'  initValue=0  dataType=int8  storage=Volatile (RAM)  calVisible=on  calType=Adjustment  calDispType=Number  calEnum={'False', 'True'}  calGain=1.0  calOffset=0  calMin=-inf  calMax=inf  calFormat='-1'  calUnit=''  calHelp=''  calAccess=1  calFunction=raptor_xcp_function(gcb)  calDispHeaders=off  calColHeaders={'Col1' 'Col2' 'Col3'}  calRowHeaders={'Row1' 'Row2' 'Row3'}
      settings: SourceProductName=Raptor
  raptor_data_write1 : Raptor_lib/Data Storage/raptor_data_write  dataName='MCU_InitFinishFlag'  dataShape=Scalar  idxSource=Input Port  idxRow=1  idxCol=1
      settings: SourceProductName=Raptor
  raptor_data_write2 : Raptor_lib/Data Storage/raptor_data_write  dataName='Rx0x701_Age'  dataShape=Scalar  idxSource=Input Port  idxRow=1  idxCol=1
      settings: SourceProductName=Raptor
  raptor_data_write3 : Raptor_lib/Data Storage/raptor_data_write  dataName='Read_MCU_Status'  dataShape=Scalar  idxSource=Input Port  idxRow=1  idxCol=1
      settings: SourceProductName=Raptor
  wires:
  raptor_can_rxmsg1/1 -> raptor_data_write2/1
  Compare To Constant/1 -> raptor_data_write1/1
  raptor_can_rxmsg1/2 -> Compare To Constant/1, raptor_data_write3/1
